simulink model "DP_Motor_with_Mass_on_Pulley"  (R2023a)
settings: Solver=VariableStepAuto  StartTime=0.0  StopTime=simtime  MaxStep=0.01  RelTol=1e-3
values from neighbouring files (symbols this model uses):
  c = 0.8    [DP_Motor_with_Mass_on_Pulley_Script.m]
  d_p_pump = 1    [DP_Motor_with_Mass_on_Pulley_Script.m]
  d_R = 1.2    [DP_Motor_with_Mass_on_Pulley_Script.m]
  eta_hm = 0.95    [DP_Motor_with_Mass_on_Pulley_Script.m]
  eta_vol = 0.95    [DP_Motor_with_Mass_on_Pulley_Script.m]
  g = 9.81    [DP_Motor_with_Mass_on_Pulley_Script.m]
  J_Mo = 5.5E-3    (= 0.0055)    [DP_Motor_with_Mass_on_Pulley_Script.m]
  k_R = 12    [DP_Motor_with_Mass_on_Pulley_Script.m]
  m = 0.6    [DP_Motor_with_Mass_on_Pulley_Script.m]
  M_L = 1.2E-2    (= 0.012)    [DP_Motor_with_Mass_on_Pulley_Script.m]
  r_D = 0.03    [DP_Motor_with_Mass_on_Pulley_Script.m]
  R_pipe = 5    [DP_Motor_with_Mass_on_Pulley_Script.m]
  V_theo = 2E-3    (= 0.002)    [DP_Motor_with_Mass_on_Pulley_Script.m]
settings Model: Creator=fycce  LastModifiedBy=fycce
settings DataIOCC: SaveOutput=off  SaveTime=off  ReturnWorkspaceOutputs=off

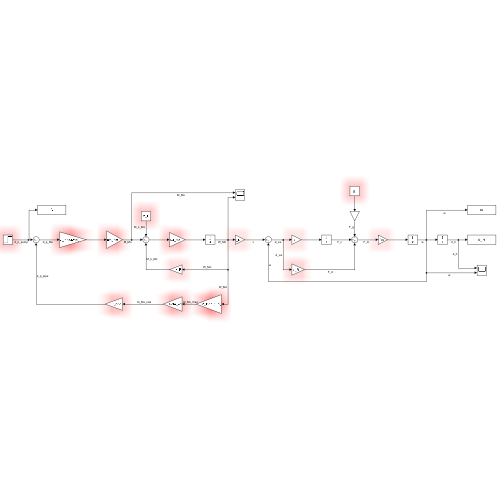
[thumbnail: Simulink's stored preview of the top-level diagram]
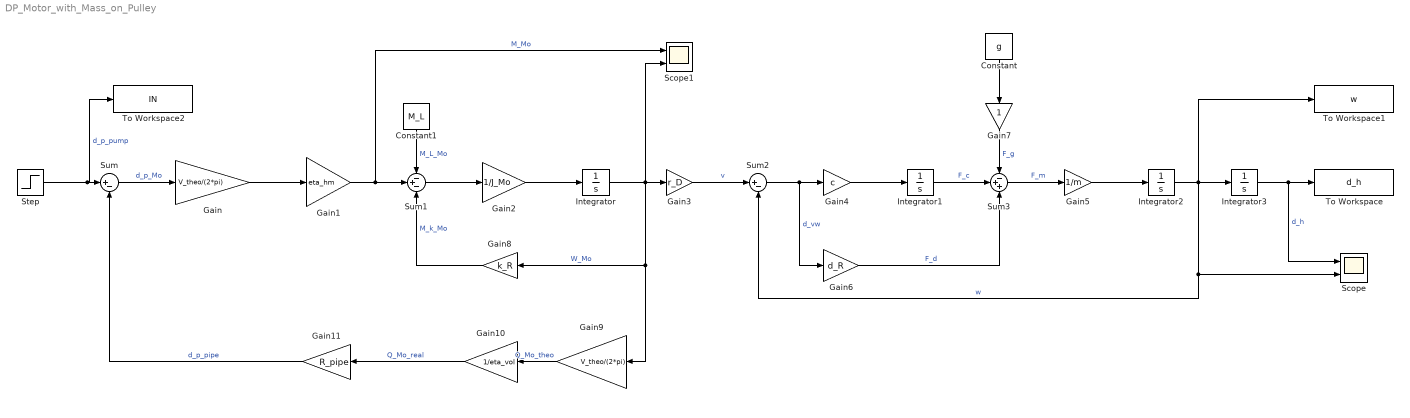
== system DP_Motor_with_Mass_on_Pulley ==
  Constant : Constant  Value=g
  Constant1 : Constant  Value=M_L
  Gain : Gain  Gain=V_theo/(2*pi)
  Gain1 : Gain  Gain=eta_hm
  Gain10 : Gain  Gain=1/eta_vol
  Gain11 : Gain  Gain=R_pipe
  Gain2 : Gain  Gain=1/J_Mo
  Gain3 : Gain  Gain=r_D
  Gain4 : Gain  Gain=c
  Gain5 : Gain  Gain=1/m
  Gain6 : Gain  Gain=d_R
  Gain7 : Gain
  Gain8 : Gain  Gain=k_R
  Gain9 : Gain  Gain=V_theo/(2*pi)
  Integrator{,1..3} (4 alike) : Integrator
  Scope : Scope  NumInputPorts=2
  Scope1 : Scope  NumInputPorts=2
  Step : Step  After=d_p_pump  SampleTime=0
  Sum : Sum  Inputs=|+-
  Sum1 : Sum  Inputs=-+-
  Sum2 : Sum  Inputs=|+-
  Sum3 : Sum  Inputs=-++
  To Workspace : ToWorkspace  VariableName=d_h  SaveFormat=Timeseries  SampleTime=-1
  To Workspace1 : ToWorkspace  VariableName=w  SaveFormat=Timeseries  SampleTime=-1
  To Workspace2 : ToWorkspace  VariableName=IN  SaveFormat=Timeseries  SampleTime=-1
  wires:
  Step/1 -> To Workspace2/1, Sum/1  "d_p_pump"
  Sum/1 -> Gain/1  "d_p_Mo"
  Gain/1 -> Gain1/1
  Gain1/1 -> Sum1/2, Scope1/1  "M_Mo"
  Sum1/1 -> Gain2/1
  Gain2/1 -> Integrator/1
  Integrator/1 -> Gain9/1, Gain8/1, Gain3/1, Scope1/2  "W_Mo"
  Gain3/1 -> Sum2/1  "v"
  Sum2/1 -> Gain4/1, Gain6/1  "d_vw"
  Gain4/1 -> Integrator1/1
  Integrator1/1 -> Sum3/2  "F_c"
  Sum3/1 -> Gain5/1  "F_m"
  Gain6/1 -> Sum3/3  "F_d"
  Gain7/1 -> Sum3/1  "F_g"
  Constant/1 -> Gain7/1
  Gain5/1 -> Integrator2/1
  Integrator2/1 -> To Workspace1/1, Sum2/2, Scope/2, Integrator3/1  "w"
  Integrator3/1 -> To Workspace/1, Scope/1  "d_h"
  Gain8/1 -> Sum1/3  "M_k_Mo"
  Constant1/1 -> Sum1/1  "M_L_Mo"
  Gain9/1 -> Gain10/1  "Q_Mo_theo"
  Gain10/1 -> Gain11/1  "Q_Mo_real"
  Gain11/1 -> Sum/2  "d_p_pipe"
